simulink model "ACDCMG_sim8"  (R2022a)
(part 10 of 12)

Yingli Energy (China) YL345D-36b | Yingli Energy (China) YL350D-36b | Yingli Energy (China) YL355D-36b | Yingli Energy (China) YL360D-36b | YOCASOL PCA200-C04 | YOCASOL PCB200-C21 | YOCASOL PCA205-C04 | YOCASOL PCB205-C21 | YOCASOL PCA210-C04 | YOCASOL PCB210-C21 | Yunnan Tianda Photovoltaic TD160M5 | Yunnan Tianda Photovoltaic TD165M5 | Yunnan Tianda Photovoltaic TD170M5 | Yunnan Tianda Photovoltaic TD175M5 | Yunnan Tianda Photovoltaic TD180M5 | Zebra Energy ZBR-185M5 | Zebra Energy ZBR-190M5 | Zebra Energy ZBR-195M5 | Zebra Energy ZBR-200M5 | Zebra Energy ZBR-200P | Zebra Energy ZBR-210P | Zebra Energy ZBR-220P | Zebra Energy ZBR-230P | Zebra Energy ZBR-235P | Zebra Energy ZBR-240MA | Zebra Energy ZBR-240PA | Zebra Energy ZBR-245MA | Zebra Energy ZBR-250MA | Zebra Energy ZBR-250P | Zebra Energy ZBR-255M | Zebra Energy ZBR-260P | Zebra Energy ZBR-270P | Zebra Energy ZBR-280P | Zebra Energy ZBR-285P | Zebra Energy ZBR-290M | Zebra Energy ZBR-290P | Zebra Energy ZBR-295M | Zebra Energy ZBR-295P | Zebra Energy ZBR-300M | Zebra Energy ZBR-300P | Zebra Energy ZBR-305M | Zebra Energy ZBR-310M | Zerquest Solar Zp170 | Zhangjiagang City SEG PV SEGM5-72 170W | Zhangjiagang City SEG PV SEGM5-72 175W | Zhangjiagang City SEG PV SEGM5-72 180W | Zhangjiagang City SEG PV SEGM5-72 185W | Zhangjiagang City SEG PV SEGM5-72 190W | Zhangjiagang City SEG PV SEGM6-54 190W | Zhangjiagang City SEG PV SEGM5-72 195W | Zhangjiagang City SEG PV SEGM6-54 195W | Zhangjiagang City SEG PV SEGM6-54 200W | Zhangjiagang City SEG PV SEGM6-60 200W | Zhangjiagang City SEG PV SEGM6-54 205W | Zhangjiagang City SEG PV SEGM6-60 205W | Zhangjiagang City SEG PV SEGM6-54 210W | Zhangjiagang City SEG PV SEGM6-60 210W | Zhangjiagang City SEG PV SEGM6-60 215W | Zhangjiagang City SEG PV SEGM6-60 220W | Zhangjiagang City SEG PV SEGM6-60 225W | Zhangjiagang City SEG PV SEGM5-96 230W | Zhangjiagang City SEG PV SEGM6-60 230W | Zhangjiagang City SEG PV SEGM5-96 235W | Zhangjiagang City SEG PV SEGM6-60 235W | Zhangjiagang City SEG PV SEGM5-96 240W | Zhangjiagang City SEG PV SEGM6-60 240W | Zhangjiagang City SEG PV SEGM5-96 245W | Zhangjiagang City SEG PV SEGM5-96 250W | Zhangjiagang City SEG PV SEGM5-96 255W | Zhangjiagang City SEG PV SEGM6-72 255W | Zhangjiagang City SEG PV SEGP6-72 255W | Zhangjiagang City SEG PV SEGM6-72 260W | Zhangjiagang City SEG PV SEGP6-72 260W | Zhangjiagang City SEG PV SEGM6-72 265W | Zhangjiagang City SEG PV SEGP6-72 265W | Zhangjiagang City SEG PV SEGM6-72 270W | Zhangjiagang City SEG PV SEGP6-72 270W | Zhangjiagang City SEG PV SEGM6-72 275W | Zhangjiagang City SEG PV SEGP6-72 275W | Zhangjiagang City SEG PV SEGM6-72 280W | Zhangjiagang City SEG PV SEGP6-72 280W | Zhangjiagang City SEG PV SEGM6-72 285W | Zhangjiagang City SEG PV SEGP6-72 285W | Zhangjiagang City SEG PV SEGM6-72 290W | Zhangjiagang City SEG PV SEGP6-72 290W | Zhangjiagang City SEG PV SEGM6-72 295W | Zhangjiagang City SEG PV SEGP6-72 295W | Zhangjiagang City SEG PV SEGM6-72 300W | Zhangjiagang City SEG PV SEGP6-72 300W | Zhangjiagang City Sunlink PV SEGP6-54-195 | Zhangjiagang City Sunlink PV SEGP6-54-200 | Zhangjiagang City Sunlink PV SEGP6-54-205 | Zhangjiagang City Sunlink PV SEGP6-60-220 | Zhangjiagang City Sunlink PV SEGP6-60-225 | Zhangjiagang City Sunlink PV SEGP6-60-230 | Zhejiang ERA Solar Technology ESPSA-170 | Zhejiang ERA Solar Technology ESPSA-175 | Zhejiang ERA Solar Technology ESPSA-180 | Zhejiang Global Photovoltaic Technology GSM-155 | Zhejiang Global Photovoltaic Technology GSM-160 | Zhejiang Global Photovoltaic Technology GSM-165 | Zhejiang Global Photovoltaic Technology GSM-170 | Zhejiang Global Photovoltaic Technology GSM-175 | Zhejiang Global Photovoltaic Technology GSM-180 | Zhejiang Global Photovoltaic Technology GSP-230 | Zhejiang Global Photovoltaic Technology GSM-235 | Zhejiang Global Photovoltaic Technology GSP-235 | Zhejiang Global Photovoltaic Technology GSM-240 | Zhejiang Global Photovoltaic Technology GSP-240 | Zhejiang Global Photovoltaic Technology GSM-245 | Zhejiang Global Photovoltaic Technology GSM-250 | Zhejiang Global Photovoltaic Technology GSP-265 | Zhejiang Global Photovoltaic Technology GSP-270 | Zhejiang Global Photovoltaic Technology GSM-275 | Zhejiang Global Photovoltaic Technology GSP-275 | Zhejiang Global Photovoltaic Technology GSM-280 | Zhejiang Global Photovoltaic Technology GSP-280 | Zhejiang Global Photovoltaic Technology GSM-285 | Zhejiang Global Photovoltaic Technology GSP-285 | Zhejiang Global Photovoltaic Technology GSM-290 | Zhejiang Global Photovoltaic Technology GSM-295 | Zhejiang Global Photovoltaic Technology GSM-300 | Zhejiang Global Photovoltaic Technology GSM-305 | Zhejiang Guangyi Optical Energy Technology GYP-150M | Zhejiang Guangyi Optical Energy Technology GYP-170P | Zhejiang Guangyi Optical Energy Technology GYP-175P | Zhejiang Guangyi Optical Energy Technology GYP-180M | Zhejiang Guangyi Optical Energy Technology GYP-180P | Zhejiang Guangyi Optical Energy Technology GYP-185M | Zhejiang Guangyi Optical Energy Technology GYP-185P | Zhejiang Guangyi Optical Energy Technology GYP-190P | Zhejiang Guangyi Optical Energy Technology GYP-200P | Zhejiang Guangyi Optical Energy Technology GYP-210P | Zhejiang Guangyi Optical Energy Technology GYP-220P | Zhejiang Guangyi Optical Energy Technology GYP-225P | Zhejiang Guangyi Optical Energy Technology GYP-230M | Zhejiang Guangyi Optical Energy Technology GYP-230P | Zhejiang Guangyi Optical Energy Technology GYP-235M | Zhejiang Guangyi Optical Energy Technology GYP-240M | Zhejiang Guangyi Optical Energy Technology GYP-245M | Zhejiang Guangyi Optical Energy Technology GYP-250M | Zhejiang Guangyi Optical Energy Technology GYP-265P | Zhejiang Guangyi Optical Energy Technology GYP-270M | Zhejiang Guangyi Optical Energy Technology GYP-270P | Zhejiang Guangyi Optical Energy Technology GYP-280M | Zhejiang Guangyi Optical Energy Technology GYP-280P | Zhejiang Guangyi Optical Energy Technology GYP-285P | Zhejiang Guangyi Optical Energy Technology GYP-290M | Zhejiang Jingshang New Energy Technology STS-6M-145P-36 | Zhejiang Jingshang New Energy Technology STS-6M-150P-36 | Zhejiang Jingshang New Energy Technology STS-6M-155P-36 | Zhejiang Jingshang New Energy Technology STS-6M-185P-48 | Zhejiang Jingshang New Energy Technology STS-6M-190P-48 | Zhejiang Jingshang New Energy Technology STS-6M-195P-48 | Zhejiang Jingshang New Energy Technology STS-6M-200P-48 | Zhejiang Jingshang New Energy Technology STS-6M-210P-54 | Zhejiang Jingshang New Energy Technology STS-6M-215P-54 | Zhejiang Jingshang New Energy Technology STS-6M-220P-54 | Zhejiang Jingshang New Energy Technology STS-6M-225P-54 | Zhejiang Jingshang New Energy Technology STS-6M-230P-54 | Zhejiang Jingshang New Energy Technology STS-6M-235P-60 | Zhejiang Jingshang New Energy Technology STS-6M-240P-60 | Zhejiang Jingshang New Energy Technology STS-6M-245P-60 | Zhejiang Jingshang New Energy Technology STS-6M-250P-60 | Zhejiang Jingshang New Energy Technology STS-6M-255P-60 | Zhejiang Jingshang New Energy Technology STS-6M-260P-60 | Zhejiang Jingshang New Energy Technology STS-6M-265P-60 | Zhejiang Jingshang New Energy Technology STS-6M-270P-72 | Zhejiang Jingshang New Energy Technology STS-6M-275P-72 | Zhejiang Jingshang New Energy Technology STS-6M-280P-72 | Zhejiang Jingshang New Energy Technology STS-6M-285P-72 | Zhejiang Jingshang New Energy Technology STS-6M-290P-72 | Zhejiang Jingshang New Energy Technology STS-6M-295P-72 | Zhejiang Jingshang New Energy Technology STS-6M-300P-72 | Zhejiang Jingshang New Energy Technology STS-6M-305P-72 | Zhejiang Jingshang New Energy Technology STS-6M-310P-72 | Zhejiang Jingshang New Energy Technology STS-6M-315P-72 | Zhejiang Jingshang New Energy Technology STS-6M-320P-72 | Zhejiang Jiutai New Energy JTM175-72M | Zhejiang Jiutai New Energy JTM180-72M | Zhejiang Jiutai New Energy JTM185-72M | Zhejiang Jiutai New Energy JTM200-60P | Zhejiang Jiutai New Energy JTM205-60P | Zhejiang Jiutai New Energy JTM210-60P | Zhejiang Jiutai New Energy JTM215-60P | Zhejiang Jiutai New Energy JTM220-60P | Zhejiang Jiutai New Energy JTM225-60P | Zhejiang Jiutai New Energy JTM230-60P | Zhejiang Jiutai New Energy JTM235-60P | Zhejiang Jiutai New Energy JTM240-60P | Zhejiang Jiutai New Energy JTM270-72P | Zhejiang Jiutai New Energy JTM275-72P | Zhejiang Jiutai New Energy JTM280-72P | Zhejiang Jiutai New Energy JTM285-72P | Zhejiang Kingdom Solar Energy Technic KD-M160 | Zhejiang Kingdom Solar Energy Technic KD-M165 | Zhejiang Kingdom Solar Energy Technic KD-M170 | Zhejiang Kingdom Solar Energy Technic KD-M175 | Zhejiang Kingdom Solar Energy Technic KD-M180 | Zhejiang Kingdom Solar Energy Technic KD-M185 | Zhejiang Kingdom Solar Energy Technic KD-M190 | Zhejiang Kingdom Solar Energy Technic KD-M195 | Zhejiang Kingdom Solar Energy Technic KD-M200 | Zhejiang Kingdom Solar Energy Technic KD-P200 | Zhejiang Kingdom Solar Energy Technic KD-P205 | Zhejiang Kingdom Solar Energy Technic KD-P210 | Zhejiang Kingdom Solar Energy Technic KD-P215 | Zhejiang Kingdom Solar Energy Technic KD-P220 | Zhejiang Kingdom Solar Energy Technic KD-P225 | Zhejiang Kingdom Solar Energy Technic KD-P230 | Zhejiang Kingdom Solar Energy Technic KD-P235 | Zhejiang Kingdom Solar Energy Technic KD-P240 | Zhejiang Kingdom Solar Energy Technic KD-P245 | Zhejiang Kingdom Solar Energy Technic KD-P250 | Zhejiang Kingdom Solar Energy Technic KD-P255 | Zhejiang Kingdom Solar Energy Technic KD-P260 | Zhejiang Kingdom Solar Energy Technic KD-P265 | Zhejiang Kingdom Solar Energy Technic KD-P270 | Zhejiang Kingdom Solar Energy Technic KD-P275 | Zhejiang Kingdom Solar Energy Technic KD-P280 | Zhejiang Kingdom Solar Energy Technic KD-P285 | Zhejiang Kingdom Solar Energy Technic KD-P290 | Zhejiang Kingdom Solar Energy Technic KD-P295 | Zhejiang Kingdom Solar Energy Technic KD-P300 | Zhejiang Shinew Photoelectronic Technology XH-72M-185 | Zhejiang Shinew Photoelectronic Technology XH-72M-190 | Zhejiang Shinew Photoelectronic Technology XH-60P-230 | Zhejiang Shinew Photoelectronic Technology XH-60P-235 | Zhejiang Shinew Photoelectronic Technology XH-72P-280 | ZheJiang SOCO Technology SC180M-24/P | ZheJiang SOCO Technology SC230M-24/J | ZheJiang SOCO Technology SC230P-24/B | ZheJiang SOCO Technology SC275P-24/A | ZheJiang SOCO Technology SC280M-24/H | Zhejiang Sunflower Light Energy Science & Technology SF125x125-72-M-150W | Zhejiang Sunflower Light Energy Science & Technology SF125x125-72-M-155W | Zhejiang Sunflower Light Energy Science & Technology SF125x125-72-M-160W | Zhejiang Sunflower Light Energy Science & Technology SF125x125-72-M-165W | Zhejiang Sunflower Light Energy Science & Technology SF125x125-72-M-170W | Zhejiang Sunflower Light Energy Science & Technology SF125x125-72-M-175W | Zhejiang Sunflower Light Energy Science & Technology SF125x125-72-M-180W | Zhejiang Sunflower Light Energy Science & Technology SF125x125-72-M-185W | Zhejiang Sunflower Light Energy Science & Technology SF156x156-60-M-200W | Zhejiang Sunflower Light Energy Science & Technology SF156x156-60-P-200W | Zhejiang Sunflower Light Energy Science & Technology SF156x156-60-M-205W | Zhejiang Sunflower Light Energy Science & Technology SF156x156-60-P-205W | Zhejiang Sunflower Light Energy Science & Technology SF156x156-60-M-210W | Zhejiang Sunflower Light Energy Science & Technology SF156x156-60-P-210W | Zhejiang Sunflower Light Energy Science & Technology SF156x156-60-M-215W | Zhejiang Sunflower Light Energy Science & Technology SF156x156-60-P-215W | Zhejiang Sunflower Light Energy Science & Technology SF156x156-60-M-220W | Zhejiang Sunflower Light Energy Science & Technology SF156x156-60-P-220W | Zhejiang Sunflower Light Energy Science & Technology SF156x156-60-M-225W | Zhejiang Sunflower Light Energy Science & Technology SF156x156-60-P-225W | Zhejiang Sunflower Light Energy Science & Technology SF156x156-60-M-230W | Zhejiang Sunflower Light Energy Science & Technology SF156x156-60-P-230W | Zhejiang Sunflower Light Energy Science & Technology SF156x156-60-M-235W | Zhejiang Sunflower Light Energy Science & Technology SF156x156-60-M-240W | Zhejiang Trunsun Solar Co._ Ltd. TSP255-60 | Zhejiang Trunsun Solar Co._ Ltd. TSM260-60 | Zhejiang Trunsun Solar Co._ Ltd. TSP260-60 | Zhejiang Trunsun Solar Co._ Ltd. TSM265-60 | Zhejiang Trunsun Solar Co._ Ltd. TSP265-60 | Zhejiang Trunsun Solar Co._ Ltd. TSM270-60 | Zhejiang Trunsun Solar Co._ Ltd. TSP270-60 | Zhejiang Trunsun Solar Co._ Ltd. TSM275-60 | Zhejiang Trunsun Solar Co._ Ltd. TSP275-60 | Zhejiang Trunsun Solar Co._ Ltd. TSP305-72 | Zhejiang Trunsun Solar Co._ Ltd. TSM310-72 | Zhejiang Trunsun Solar Co._ Ltd. TSP310-72 | Zhejiang Trunsun Solar Co._ Ltd. TSM315-72 | Zhejiang Trunsun Solar Co._ Ltd. TSP315-72 | Zhejiang Trunsun Solar Co._ Ltd. TSM320-72 | Zhejiang Trunsun Solar Co._ Ltd. TSP320-72 | Zhejiang Trunsun Solar Co._ Ltd. TSM325-72 | Zhejiang Trunsun Solar Co._ Ltd. TSP325-72 | Zhejiang Trunsun Solar Co._ Ltd. TSM330-72 | Zhejiang Trunsun Solar Co._ Ltd. TSP330-72 | Zhejiang Trunsun Solar Co._ Ltd. TSP335-72 | Zhejiang Wanxiang Solar WXS175P | Zhejiang Wanxiang Solar WXS175S | Zhejiang Wanxiang Solar WXS180P | Zhejiang Wanxiang Solar WXS180S | Zhejiang Wanxiang Solar WXS185P | Zhejiang Wanxiang Solar WXS185S | Zhejiang Wanxiang Solar WXS190P | Zhejiang Wanxiang Solar WXS200P | Zhejiang Wanxiang Solar WXS205P | Zhejiang Wanxiang Solar WXS210P | Zhejiang Wanxiang Solar WXS215P | Zhejiang Wanxiang Solar WXS220P | Zhejiang Wanxiang Solar WXS225P | Zhejiang Wanxiang Solar WXS230P | Zhejiang Wanxiang Solar WXS235P | Zhejiang Wanxiang Solar WXS240P | Zhejiang Wanxiang Solar WXS245P | Zhejiang Wanxiang Solar WXS250P | Zhejiang Wanxiang Solar WXS255P | Zhejiang Wanxiang Solar WXS260P | Zhejiang Wanxiang Solar WXS265P | Zhejiang Wanxiang Solar WXS270P | Zhejiang Wanxiang Solar WXS275P | Zhejiang Wanxiang Solar WXS280P | Znshine PV-Tech ZXM5-72-175/MS | Znshine PV-Tech ZXM5-72-180/MS | Znshine PV-Tech ZXM5-72-185/MS | Znshine PV-Tech ZXM5-72-190/MS | Znshine PV-Tech ZXM5-72-195/MS | Znshine PV-Tech ZXM5-72-200/MS | Znshine PV-Tech ZXP6-60-220/P | Znshine PV-Tech ZXP6-60-225/P | Znshine PV-Tech ZXP6-60-230/P | Znshine PV-Tech ZXP6-60-235/P | Znshine PV-Tech ZXP6-D60-235/P | Znshine PV-Tech ZXM6-D60-240/M | Znshine PV-Tech ZXP6-60-240/P | Znshine PV-Tech ZXP6-D60-240/P | Znshine PV-Tech ZXM5-96-245/MS | Znshine PV-Tech ZXM6-D60-245/M | Znshine PV-Tech ZXP6-60-245/P | Znshine PV-Tech ZXP6-D60-245/P | Znshine PV-Tech ZXM5-96-250/MS | Znshine PV-Tech ZXM6-D60-250/M | Znshine PV-Tech ZXP6-D60-250/P | Znshine PV-Tech ZXM5-96-255/MS | Znshine PV-Tech ZXM6-D60-255/M | Znshine PV-Tech ZXP6-D60-255/P | Znshine PV-Tech ZXM5-96-260/MS | Znshine PV-Tech ZXM6-D60-260/M | Znshine PV-Tech ZXM5-96-265/MS | Znshine PV-Tech ZXP6-72-265/P | Znshine PV-Tech ZXM5-96-270/MS | Znshine PV-Tech ZXP6-72-270/P | Znshine PV-Tech ZXM5-96-275/MS | Znshine PV-Tech ZXP6-72-275/P | Znshine PV-Tech ZXP6-72-280/P | Znshine PV-Tech ZXP6-72-285/P | Znshine PV-Tech ZXP6-72-290/P | Znshine PV-Tech ZXP6-72-295/P | Zytech Engineering Technology ZT170S | Zytech Engineering Technology ZT175S | Zytech Engineering Technology ZT180S | Zytech Engineering Technology ZT185S | Zytech Engineering Technology ZT190S | Zytech Solar ZT145P | Zytech Solar ZT150P | Zytech Solar ZT155P | Zytech Solar ZT185P | Zytech Solar ZT190P | Zytech Solar ZT195P | Zytech Solar ZT200P | Zytech Solar ZT210P | Zytech Solar ZT215P | Zytech Solar ZT220P | Zytech Solar ZT225P | Zytech Solar ZT230P | Zytech Solar ZT235P | Zytech Solar ZT240P | Zytech Solar ZT245P | Zytech Solar ZT250P | Zytech Solar ZT255P | Zytech Solar ZT260P | Zytech Solar ZT265P | Zytech Solar ZT270P | Zytech Solar ZT275P | Zytech Solar ZT280P | Zytech Solar ZT285P | Zytech Solar ZT290P | Zytech Solar ZT295P | Zytech Solar ZT300P | Zytech Solar ZT305P | Zytech Solar ZT310P | Zytech Solar ZT315P | Zytech Solar ZT320P
      mask Callback ModuleName: PVArrayCback(gcb)
      mask Callback RobustModel: PVArrayCback(gcb)
      mask Callback BAL: PVArrayCback(gcb)
      mask DialogControl ParameterTabVar0 Prompt: Parameters
      mask DialogControl ArrayData Prompt: Array data
      mask DialogControl Display Prompt: Display  I-V and P-V characteristics of ...
      mask DialogControl PlotButton Prompt: Plot
      mask DialogControl PlotButton Callback: PVArrayPlot(gcb,'detailed')
      mask DialogControl ManufacturerData Prompt: Module data
      mask DialogControl ModelParameters Prompt: Model parameters
      mask DialogControl Advanced Prompt: Advanced
      mask Display:
      | port_label('input',1,'Ir')
      | switch WantBlockChoice{1}
      |     case 'Discrete DSS Diode Rsh'
      |     otherwise
      |         port_label('input',2,'T')
      | end
      | 
      | port_label('output',1,'m')
      | port_label('output',1,'m')
      | port_label('Rconn',1,'+')
      | port_label('Rconn',2,'-')
  Scope : Scope  NumInputPorts=2
  Temp C : Constant  Value=25
  V : spsVoltageMeasurementLib/Voltage Measurement  PhasorSimulation=off  OutputType=Complex  PSBequivalent=0
  T2+ : PMIOPort  Side=Right
  T2- : PMIOPort  Port=2  Side=Right
  tag scope: m_PV=global
  wires:
  V/1 -> Scope/2, [V]
  Diode1/1 -> [VI_D]
  Temp C/1 -> PV Panel/2(TempC)
  PV Panel/1(m) -> [m_PV], Bus Selector/1
  Ir1/1 -> PV Panel/1(S)
  Bus Selector/1 -> [VI_PV]
  I/1 -> Scope/1, [I]
  connections:
  V/LConn1 -- I/LConn1 -- PV Panel/RConn1 -- Diode1/RConn1
  T2-/RConn1 -- V/LConn2 -- Diode1/LConn1 -- PV Panel/RConn2
  I/RConn1 -- T2+/RConn1
